simulink model "PID_ROVNonLinearModel"  (R2024a)
settings: Solver=VariableStepAuto  StartTime=0.0  StopTime=200  RelTol=1e-3
libraries: slpidlib x1
settings Model: Creator=Shiva  LastModifiedBy=root
settings ModelReferenceCC: EnableRefExpFcnMdlSchedulingChecks=on
settings RTWCC: GPUComputeCapability=3.5

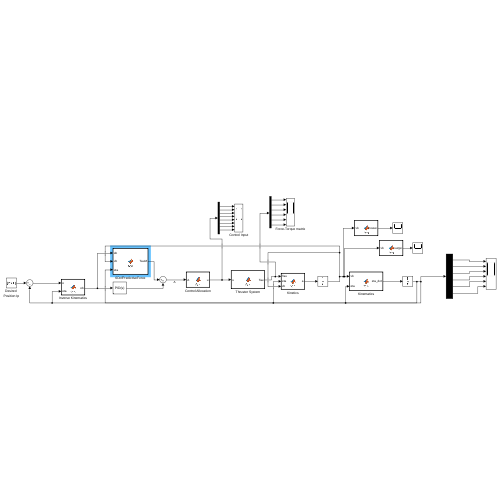
[thumbnail: Simulink's stored preview of the top-level diagram]
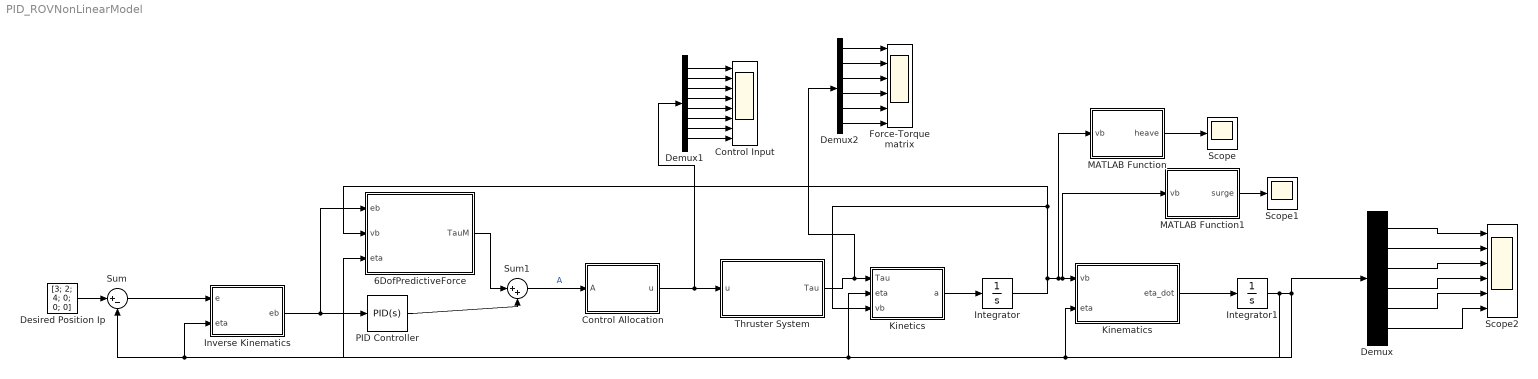
== system PID_ROVNonLinearModel ==
  6DofPredictiveForce : MATLAB Function  TreatAsAtomicUnit=on
  Control Allocation : MATLAB Function  TreatAsAtomicUnit=on
  Control Input : Scope  NumInputPorts=8
  Demux : Demux  Outputs=6
  Demux1 : Demux  Outputs=8
  Demux2 : Demux  Outputs=6
  Desired Position Ip : Constant  Value=[3; 2; 4; 0; 0; 0]
  Force-Torque matrix : Scope  NumInputPorts=6
  Integrator : Integrator  InitialCondition=[0;0;0;0;0;0]
  Integrator1 : Integrator  InitialCondition=[0;0;0;0;0;0]
  Inverse Kinematics : MATLAB Function  TreatAsAtomicUnit=on
  Kinematics : MATLAB Function  TreatAsAtomicUnit=on
  Kinetics : MATLAB Function  TreatAsAtomicUnit=on
  MATLAB Function : MATLAB Function  TreatAsAtomicUnit=on
  MATLAB Function1 : MATLAB Function  TreatAsAtomicUnit=on
  PID Controller : slpidlib/PID Controller  Controller=PID  Form=Parallel  TimeDomain=Continuous-time  UseExternalTs=off  SampleTime=-1  IntegratorMethod=Forward Euler  FilterMethod=Forward Euler  ControllerParametersSource=internal  P=[1;1;1.2;0.3;0.3;0.3]  I=[0.001; 0.001; 0.001; 0.001; 0.001; 0.001]  UseKiTs=off  D=[0; 0; 1.5; 0.3; 0.3; 0.3]  UseExternalDerivativeSource=off  N=100  UseFilter=on  TunerSelectOption=Frequency Response Based  InitialConditionSource=internal  InitialConditionForIntegrator=[0;0;0;0;0;0]  InitialConditionForFilter=[0;0;0;0;0;0]  DifferentiatorICPrevScaledInput=0  ExternalReset=none  TrackingMode=off  Kt=1  LimitOutput=off  SatLimitsSource=internal  UpperSaturationLimit=inf  LowerSaturationLimit=-inf  LinearizeAsGain=on  AntiWindupMode=none  Kb=1  LimitIntegrator=off  UpperIntegratorSaturationLimit=inf  LowerIntegratorSaturationLimit=-inf  POutMin=[]  POutMax=[]  IOutMin=[]  IOutMax=[]  DOutMin=[]  DOutMax=[]  NOutMin=[]  NOutMax=[]  SumOutMin=[]  SumOutMax=[]  SaturationOutMin=[]  SaturationOutMax=[]  PParamMin=[]  PParamMax=[]  IParamMin=[]  IParamMax=[]  DParamMin=[]  DParamMax=[]  NParamMin=[]  NParamMax=[]  KbParamMin=[]  KbParamMax=[]  KtParamMin=[]  KtParamMax=[]  KbOutMin=[]  KbOutMax=[]  KtOutMin=[]  KtOutMax=[]  IntegratorOutMin=[]  IntegratorOutMax=[]  FilterOutMin=[]  FilterOutMax=[]  SumI1OutMin=[]  SumI1OutMax=[]  SumI2OutMin=[]  SumI2OutMax=[]  SumI3OutMin=[]  SumI3OutMax=[]  SumI4OutMin=[]  SumI4OutMax=[]  SumDOutMin=[]  SumDOutMax=[]  DifferentiatorOutMin=[]  DifferentiatorOutMax=[]  FilterDiffOutCoefMin=[]  FilterDiffOutCoefMax=[]  ReciprocalOutMin=[]  ReciprocalOutMax=[]  SumDenOutMin=[]  SumDenOutMax=[]  SumNumOutMin=[]  SumNumOutMax=[]  DivideOutMin=[]  DivideOutMax=[]  UdiffTsProdOutMin=[]  UdiffTsProdOutMax=[]  NTsProdOutMin=[]  NTsProdOutMax=[]  UintegralTsProdOutMin=[]  UintegralTsProdOutMax=[]  UngainTsProdOutMin=[]  UngainTsProdOutMax=[]  ClampingZeroOutDataTypeStr=Inherit: Inherit via back propagation  ClampingZeroOutMin=[]  ClampingZeroOutMax=[]  FilterDenConstantOutDataTypeStr=Inherit: Inherit via back propagation  FilterDenConstantOutMin=[]  FilterDenConstantOutMax=[]  PCopyOutDataTypeStr=Inherit: Inherit via back propagation  PCopyOutMin=[]  PCopyOutMax=[]  NCopyOutDataTypeStr=Inherit: Inherit via back propagation  NCopyOutMin=[]  NCopyOutMax=[]  IntegratorContinuousStateAttributes=''  IntegratorStateMustResolveToSignalObject=off  IntegratorRTWStateStorageClass=Auto  FilterContinuousStateAttributes=''  FilterStateMustResolveToSignalObject=off  FilterRTWStateStorageClass=Auto  ParallelPVariant=InternalParameters  IdealPVariant=Disabled  IVariant=InternalParameters  DVariant=InternalParameters  IntegratorVariant=Continuous  SatVariant=Disabled  AWVariant=Passthrough  PCopyVariant=Disabled  TRVariant=Disabled  FdbkBlocksVariant=Forward  IdealPFdbkVariant=Disabled  SatFdbkVariant=Disabled  DerivativeFilterVariant=ContFilter  NVariant=InternalParameters  NCopyVariant=Disabled  FilterICVariant=InternalICsFilter  IntegratorICVariant=InternalICs  ExternalResetVariant=Disabled  TRSumVariant=Passthrough  SumFdbkVariant=Disabled  SumVariant=Sum_PID  TsampFilterVariant=InternalTs  TsampNgainVariant=Passthrough  TsampIntegralVariant=Disabled_SignalSpec  ExternalSaturationOutDataTypeStr=Inherit: Same as second input  DerivativeSourceVariant=ErrorSignal
  Scope : Scope
  Scope1 : Scope
  Scope2 : Scope  NumInputPorts=6
  Sum : Sum  Inputs=|+-
  Sum1 : Sum  Inputs=|++
  Thruster System : MATLAB Function  TreatAsAtomicUnit=on
  wires:
  Thruster System/1(Tau) -> Demux2/1, Kinetics/1(Tau)
  Kinetics/1(a) -> Integrator/1
  Integrator/1 -> Kinetics/3(vb), 6DofPredictiveForce/2(vb), MATLAB Function/1(vb), MATLAB Function1/1(vb), Kinematics/1(vb)
  Kinematics/1(eta_dot) -> Integrator1/1
  Integrator1/1 -> 6DofPredictiveForce/3(eta), Demux/1, Inverse Kinematics/2(eta), Sum/2, Kinetics/2(eta), Kinematics/2(eta)
  Sum/1 -> Inverse Kinematics/1(e)
  Inverse Kinematics/1(eb) -> 6DofPredictiveForce/1(eb), PID Controller/1
  Sum1/1 -> Control Allocation/1(A)  "A"
  Control Allocation/1(u) -> Demux1/1, Thruster System/1(u)
  6DofPredictiveForce/1(TauM) -> Sum1/1
  PID Controller/1 -> Sum1/2
  Desired Position Ip/1 -> Sum/1
  Demux1/1 -> Control Input/1
  Demux1/2 -> Control Input/2
  Demux1/3 -> Control Input/3
  Demux1/4 -> Control Input/4
  Demux1/5 -> Control Input/5
  Demux1/6 -> Control Input/6
  Demux2/1 -> Force-Torque matrix/1
  Demux2/3 -> Force-Torque matrix/3
  Demux2/5 -> Force-Torque matrix/5
  Demux2/2 -> Force-Torque matrix/2
  Demux2/6 -> Force-Torque matrix/6
  Demux2/4 -> Force-Torque matrix/4
  Demux1/7 -> Control Input/7
  Demux1/8 -> Control Input/8
  MATLAB Function/1(heave) -> Scope/1
  MATLAB Function1/1(surge) -> Scope1/1
  Demux/1 -> Scope2/1
  Demux/2 -> Scope2/2
  Demux/3 -> Scope2/3
  Demux/4 -> Scope2/4
  Demux/5 -> Scope2/5
  Demux/6 -> Scope2/6

== matlab function PID_ROVNonLinearModel/Thruster System ==
  data: u input; Tau output
function Tau = fcn(u)

T=[0.707,0.707,-0.707,-0.707,0,0,0,0;
   -0.707,0.707,-0.707,0.707,0,0,0,0;
   0,0,0,0,-1,1,1,-1;
   0.06,-0.06,0.06,-0.06,-0.218,-0.218,0.218,0.218;
   0.06,0.06,-0.06,-0.06,0.120,-0.120,0.120,-0.120;
   -0.1888,0.1888,0.1888,-0.1888,0,0,0,0];

K=diag([40,40,40,40,40,40,40,40]);

%T_star=(T.')*inv(T*(T.'));

Tau=T*(K*u);

== matlab function PID_ROVNonLinearModel/Kinematics ==
  data: vb input; eta_dot output; eta input
function eta_dot = fcn(vb,eta)
phi=eta(4);
theta=eta(5);
psi=eta(6);
R=[cos(psi)*cos(theta),-sin(psi)*cos(phi)+cos(psi)*sin(theta)*sin(phi),sin(psi)*sin(phi)+cos(psi)*cos(phi)*sin(theta);
    sin(psi)*cos(theta),cos(psi)*cos(phi)+sin(psi)*sin(theta)*sin(phi),-cos(psi)*sin(phi)+sin(theta)*sin(psi)*cos(phi);
    -sin(theta),cos(theta)*sin(phi),cos(theta)*cos(phi)];

T=[1,sin(phi)*tan(theta),cos(phi)*tan(theta);
    0,cos(phi),-sin(phi);
    0,sin(phi)/cos(theta),cos(phi)/cos(theta)];

J=[R,zeros(3,3);zeros(3,3),T];

eta_dot=J*vb;

== matlab function PID_ROVNonLinearModel/Inverse Kinematics ==
  data: e input; eb output; eta input
function eb = fcn(e,eta)
phi=eta(4);
theta=eta(5);
psi=eta(6);
R=[cos(psi)*cos(theta),-sin(psi)*cos(phi)+cos(psi)*sin(theta)*sin(phi),sin(psi)*sin(phi)+cos(psi)*cos(phi)*sin(theta);
    sin(psi)*cos(theta),cos(psi)*cos(phi)+sin(psi)*sin(theta)*sin(phi),-cos(psi)*sin(phi)+sin(theta)*sin(psi)*cos(phi);
    -sin(theta),cos(theta)*sin(phi),cos(theta)*cos(phi)];

T=[1,sin(phi)*tan(theta),cos(phi)*tan(theta);
    0,cos(phi),-sin(phi);
    0,sin(phi)/cos(theta),cos(phi)/cos(theta)];

J=[R,zeros(3,3);zeros(3,3),T];

eb=(J.')*e;

== matlab function PID_ROVNonLinearModel/6DofPredictiveForce ==
  data: eb input; TauM output; vb input; eta input
function TauM = fcn(eb,vb,eta)
phi=eta(4);
theta=eta(5);
%psi=eta(6);
u=vb(1);
v=vb(2);
w=vb(3);
p=vb(4);
q=vb(5);
r=vb(6);
m=11.5;
zg=0.02;
Ix=0.6;
Iy=0.6;
Iz=0.6;
W=112.8;
B=114.8;
M=[m,0,0,0,m*zg,0;
    0,m,0,-m*zg,0,0;
    0,0,m,0,0,0;
    0,-m*zg,0,Ix,0,0;
    m*zg,0,0,0,Iy,0;
    0,0,0,0,0,Iz
    ];
MA=diag([5.5,12.7,14.57,0.12,0.12,0.12]);
Meff=M+MA;
vc=[0.1;0.1;0;0;0;0];
CRB=[0,0,0,0,m*w,0;
    0,0,0,-m*w,0,0;
    0,0,0,m*v,-m*u,0;
    0,m*w,-m*v,0,Iz*r,-Iy*q;
    -m*w,0,-m*u,-Iz*r,0,Ix*p;
    m*v,-m*u,0,Iy*q,-Ix*p,0];
CA=[0,0,0,0,-14.57*w,0;
    0,0,0,14.57*w,0,5.5*u;
    0,0,0,12.7*v,-5.5*u,0;
    0,14.57*w,-12.7*v,0,0.12*r,-0.12*q;
    -14.57*w,0,5.5*u,-0.12*r,0,0.12*p;
    12.57*v,-5.5*u,0,0.12*q,-0.12*p,0
    ];
D=diag([4.03+18.18*abs(u),6.22+21.66*abs(v),5.18+36.99*abs(w),0.07+1.55*abs(p),0.07+1.55*abs(q),0.07+1.55*abs(r)]);
g=[(W-B)*sin(theta);-(W-B)*cos(theta)*sin(phi);-(W-B)*cos(theta)*cos(phi);zg*W*cos(theta)*sin(phi);zg*W*sin(theta);0];

vd=[0.4;0.4;0;0;0;0];
vd_dot=[0;0;0;0;0;0];
lambda=[0.1;0.1;0.001;0.1;0.1;0.1];

TauM=Meff*(vd_dot+lambda.*(vd-vb))+CRB*vb+CA*(vb-vc)+D*(vd+lambda.*eb-vc)+g;

== matlab function PID_ROVNonLinearModel/Control Allocation ==
  data: A input; u output
function u = fcn(A)
T=[0.707,0.707,-0.707,-0.707,0,0,0,0;
   -0.707,0.707,-0.707,0.707,0,0,0,0;
   0,0,0,0,-1,1,1,-1;
   0.06,-0.06,0.06,-0.06,-0.218,-0.218,0.218,0.218;
   0.06,0.06,-0.06,-0.06,0.120,-0.120,0.120,-0.120;
   -0.1888,0.1888,0.1888,-0.1888,0,0,0,0];

K=diag([40,40,40,40,40,40,40,40]);

T_star=(T.')*inv(T*(T.'));

u=inv(K)*T_star*A;

== matlab function PID_ROVNonLinearModel/MATLAB Function ==
  data: vb input; heave output
function heave = fcn(vb)
heave=vb(3);

== matlab function PID_ROVNonLinearModel/MATLAB Function1 ==
  data: vb input; surge output
function surge = fcn(vb)
surge=vb(1);

== matlab function PID_ROVNonLinearModel/Kinetics ==
  data: Tau input; a output; eta input; vb input
function a = fcn(Tau,eta,vb)

phi=eta(4);
theta=eta(5);
%psi=eta(6);
u=vb(1);
v=vb(2);
w=vb(3);
p=vb(4);
q=vb(5);
r=vb(6);
m=11.5;
W=112.8;
B=114.8;
Ix=0.16;
Iy=0.16;
Iz=0.16;
zg=0.02;
M=[m,0,0,0,m*zg,0;
    0,m,0,-m*zg,0,0;
    0,0,m,0,0,0;
    0,-m*zg,0,Ix,0,0;
    m*zg,0,0,0,Iy,0;
    0,0,0,0,0,Iz
    ];
MA=diag([5.5,12.7,14.57,0.12,0.12,0.12]);
Meff=M+MA;
vc=[0.1;0.1;0;0;0;0];
CRB=[0,0,0,0,m*w,0;
    0,0,0,-m*w,0,0;
    0,0,0,m*v,-m*u,0;
    0,m*w,-m*v,0,Iz*r,-Iy*q;
    -m*w,0,-m*u,-Iz*r,0,Ix*p;
    m*v,-m*u,0,Iy*q,-Ix*p,0];
CA=[0,0,0,0,-14.57*w,0;
    0,0,0,14.57*w,0,5.5*u;
    0,0,0,12.7*v,-5.5*u,0;
    0,14.57*w,-12.7*v,0,0.12*r,-0.12*q;
    -14.57*w,0,5.5*u,-0.12*r,0,0.12*p;
    12.57*v,-5.5*u,0,0.12*q,-0.12*p,0
    ];
D=diag([4.03+18.18*abs(u),6.22+21.66*abs(v),5.18+36.99*abs(w),0.07+1.55*abs(p),0.07+1.55*abs(q),0.07+1.55*abs(r)]);
g=[(W-B)*sin(theta);-(W-B)*cos(theta)*sin(phi);-(W-B)*cos(theta)*cos(phi);zg*W*cos(theta)*sin(phi);zg*W*sin(theta);0];

a=inv(Meff)*(Tau-CRB*vb-CA*(vb-vc)-D*(vb-vc)-g);
